simulink model "TASK_1"  (R2018b)
settings: Solver=VariableStepAuto  StartTime=0.0  StopTime=40  MaxStep=1e-5  RelTol=1e-3
settings Model: Creator=STUDENT  LastModifiedBy=Федор
settings SFSimCC: SimUseLocalCustomCode=off
settings RTWCC: RTWUseLocalCustomCode=off
settings CodeAppCC: StateflowObjectComments=on
settings SimscapeCC: SimscapeNormalizeSystem=off

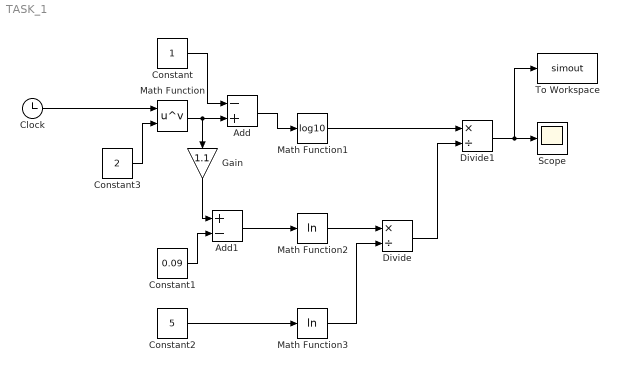
== system TASK_1 ==
  Add : Sum  Inputs=-+
  Add1 : Sum  Inputs=+-
  Clock : Clock
  Constant : Constant
  Constant1 : Constant  Value=0.09
  Constant2 : Constant  Value=5
  Constant3 : Constant  Value=2
  Divide : Product  Inputs=*/
  Divide1 : Product  Inputs=*/
  Gain : Gain  Gain=1.1
  Math Function : Math  Operator=pow  SaturateOnIntegerOverflow=on
  Math Function1 : Math  Operator=log10  SaturateOnIntegerOverflow=on
  Math Function2 : Math  Operator=log  SaturateOnIntegerOverflow=on
  Math Function3 : Math  Operator=log  SaturateOnIntegerOverflow=on
  Scope : Scope
  To Workspace : ToWorkspace  VariableName=simout  SaveFormat=Timeseries  SampleTime=-1
  wires:
  Clock/1 -> Math Function/1
  Add/1 -> Math Function1/1
  Constant1/1 -> Add1/2
  Gain/1 -> Add1/1
  Add1/1 -> Math Function2/1
  Constant2/1 -> Math Function3/1
  Math Function2/1 -> Divide/1
  Math Function3/1 -> Divide/2
  Math Function1/1 -> Divide1/1
  Divide/1 -> Divide1/2
  Divide1/1 -> Scope/1, To Workspace/1
  Constant3/1 -> Math Function/2
  Math Function/1 -> Gain/1, Add/2
  Constant/1 -> Add/1
